simulink model "matrice_forces_centrifuges"  (R2022b)
settings: Solver=VariableStepAuto  StartTime=0.0  StopTime=10.0  RelTol=1e-3
undefined symbols (not defined in the file): l1, l2, m2
settings Model: Creator=cheye  LastModifiedBy=cheye

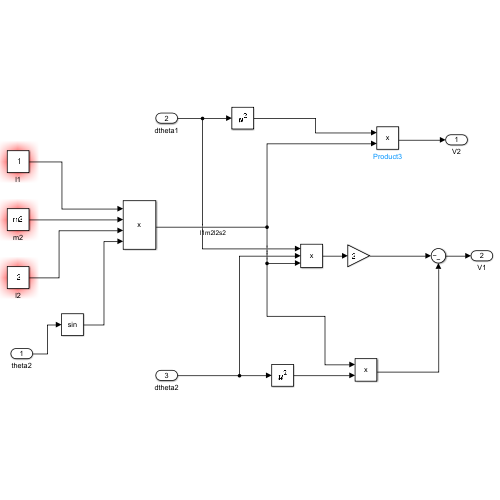
[thumbnail: Simulink's stored preview of the top-level diagram]
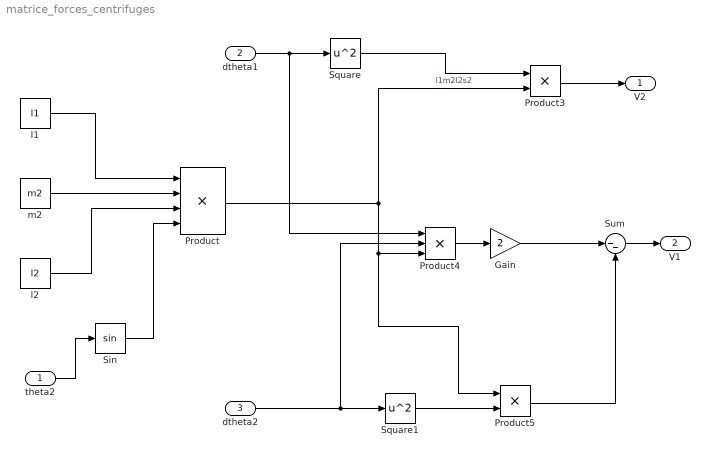
== system matrice_forces_centrifuges ==
  theta2 : Inport
  dtheta1 : Inport  Port=2
  dtheta2 : Inport  Port=3
  Gain : Gain  Gain=2
  Product : Product  Inputs=4
  Product3 : Product
  Product4 : Product  Inputs=3
  Product5 : Product
  Sin : Trigonometry
  Square : Math  Operator=square
  Square1 : Math  Operator=square
  Sum : Sum  Inputs=|--
  l1 : Constant  Value=l1
  l2 : Constant  Value=l2
  m2 : Constant  Value=m2
  V2 : Outport
  V1 : Outport  Port=2
  wires:
  l1/1 -> Product/1
  m2/1 -> Product/2
  dtheta1/1 -> Product4/1, Square/1
  Square/1 -> Product3/1
  l2/1 -> Product/3
  Product/1 -> Product4/3, Product5/1, Product3/2  "l1m2l2s2"
  dtheta2/1 -> Square1/1, Product4/2
  Product3/1 -> V2/1
  Square1/1 -> Product5/2
  Product4/1 -> Gain/1
  Gain/1 -> Sum/1
  Product5/1 -> Sum/2
  Sum/1 -> V1/1
  theta2/1 -> Sin/1
  Sin/1 -> Product/4
